simulink model "six_step_inverter"  (R2023b)
settings: Solver=VariableStepAuto  StartTime=0.0  StopTime=2  RelTol=1e-3
libraries: spsIGBTDiodeLib x6, spsSeriesRLCBranchLib x3, spsDCVoltageSourceLib x1, spsGroundLib x1, spsMultimeterLib x1, sps_lib x1
settings Model: Creator=lmanglicmot  LastModifiedBy=lmanglicmot
settings DataIOCC: ReturnWorkspaceOutputs=off
settings OptimizationCC: ReuseModelBlockBuffer=off

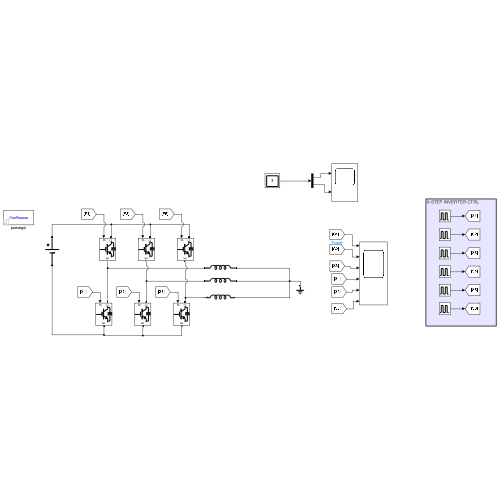
[thumbnail: Simulink's stored preview of the top-level diagram]
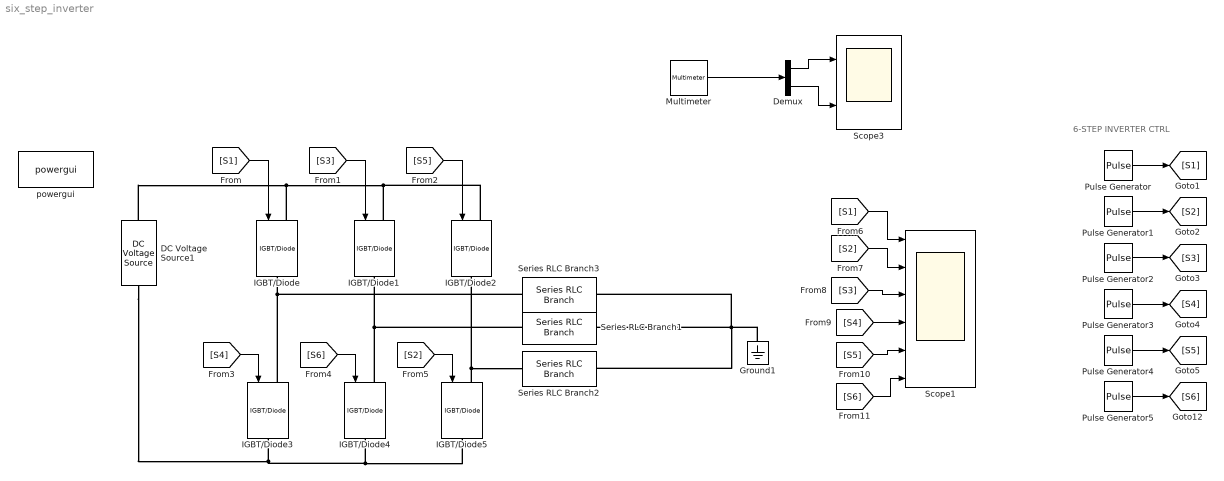
== system six_step_inverter ==
  note: 6-STEP INVERTER CTRL
  DC Voltage Source1 : spsDCVoltageSourceLib/DC Voltage Source  Amplitude=50  Measurements=None
  Demux : Demux  Outputs=2
  Ground1 : spsGroundLib/Ground  LConnTagsString=a
  IGBT/Diode{,1..5} (6 alike) : spsIGBTDiodeLib/IGBT//Diode  Ron=1e-3  Rs=1e5  Cs=inf  Measurements=off
  Multimeter : spsMultimeterLib/Multimeter  L=3  sel=[1 2 3]  yselected={}  Gain=[1 1 1]  OutputType=Complex  PlotAtSimulationStop=off  PhasorSimulation=off
  Pulse Generator : DiscretePulseGenerator  PulseType=Time based  Period=1/60  PulseWidth=50%
  Pulse Generator1 : DiscretePulseGenerator  PulseType=Time based  Period=1/60  PulseWidth=50%  PhaseDelay=(1/6)*1/60
  Pulse Generator2 : DiscretePulseGenerator  PulseType=Time based  Period=1/60  PulseWidth=50%  PhaseDelay=(2/6)*1/60
  Pulse Generator3 : DiscretePulseGenerator  PulseType=Time based  Period=1/60  PulseWidth=50  PhaseDelay=(3/6)*1/60
  Pulse Generator4 : DiscretePulseGenerator  PulseType=Time based  Period=1/60  PulseWidth=50%  PhaseDelay=(4/6)*1/60
  Pulse Generator5 : DiscretePulseGenerator  PulseType=Time based  Period=1/60  PulseWidth=50%  PhaseDelay=(5/6)*1/60
  Scope1 : Scope  NumInputPorts=6
  Scope3 : Scope  NumInputPorts=2
  Series RLC Branch1 : spsSeriesRLCBranchLib/Series RLC Branch  LConnTagsString=__new0  RConnTagsString=__new0  BranchType=L  Resistance=1  Inductance=5e-3  SetiL0=off  InitialCurrent=0  Capacitance=1e-6  Setx0=off  InitialVoltage=0  Measurements=Branch voltage
  Series RLC Branch2 : spsSeriesRLCBranchLib/Series RLC Branch  LConnTagsString=__new0  RConnTagsString=__new0  BranchType=L  Resistance=1  Inductance=5e-3  SetiL0=off  InitialCurrent=0  Capacitance=1e-6  Setx0=off  InitialVoltage=0  Measurements=Branch voltage
  Series RLC Branch3 : spsSeriesRLCBranchLib/Series RLC Branch  LConnTagsString=__new0  RConnTagsString=__new0  BranchType=L  Resistance=1  Inductance=5e-3  SetiL0=off  InitialCurrent=0  Capacitance=1e-6  Setx0=off  InitialVoltage=0  Measurements=Branch voltage
  powergui : sps_lib/powergui  Priority=1  SimulationMode=Continuous  SampleTime=1e-6  frequency=60  Iterations=50  frequencyindice=0  Pbase=100e6  ErrMax=1e-4  UnitsV=kV  UnitsW=MW  buscounter=0  FunctionMessages=off  echomessages=off  EnableUseOfTLC=off  CurrentSourceSwitches=off  DisableSnubberDevices=off  DisableRonSwitches=off  DisableVfSwitches=off  DisplayEquations=off  AutomaticDiscreteSolvers=off  SolverType=Tustin/Backward Euler (TBE)  Interpol=off  ExternalGateDelay=off  methode=off  Ts=100  x0status=blocks  SPID=on  SwTol=0  HookPort=off  NonlinearTolerance=1e-4  nMaxIteration=100  ContinueOnMaxIteration=off  RestoreLinks=warning  ResistiveCurrentMeasurement=off  Frange=[0:2:500]  Ylog=off  Xlog=on  ShowGrid=off  save=off  variable=ZData  structure=0  ZoomFFT=off  StartTime=0.0  cycles=1  DisplayStyle=1  fundamental=60  FreqAxis=off  MaxFrequency=1000  frequencyindicesteady=1  RmsSteady=1  display=off
  wires:
  [S1] -> IGBT/Diode/1
  [S3] -> IGBT/Diode1/1
  [S5] -> IGBT/Diode2/1
  [S4] -> IGBT/Diode3/1
  [S6] -> IGBT/Diode4/1
  [S2] -> IGBT/Diode5/1
  Pulse Generator/1 -> [S1]
  Pulse Generator1/1 -> [S2]
  Pulse Generator2/1 -> [S3]
  Pulse Generator3/1 -> [S4]
  Pulse Generator4/1 -> [S5]
  Pulse Generator5/1 -> [S6]
  [S1] -> Scope1/1
  [S2] -> Scope1/2
  [S3] -> Scope1/3
  [S4] -> Scope1/4
  [S5] -> Scope1/5
  [S6] -> Scope1/6
  Multimeter/1 -> Demux/1
  Demux/1 -> Scope3/1
  Demux/2 -> Scope3/2
  connections:
  Series RLC Branch3/LConn1 -- IGBT/Diode/RConn1 -- IGBT/Diode3/LConn1
  IGBT/Diode4/LConn1 -- IGBT/Diode1/RConn1 -- Series RLC Branch1/LConn1
  IGBT/Diode5/LConn1 -- IGBT/Diode2/RConn1 -- Series RLC Branch2/LConn1
  IGBT/Diode/LConn1 -- DC Voltage Source1/RConn1 -- IGBT/Diode2/LConn1 -- IGBT/Diode1/LConn1
  IGBT/Diode5/RConn1 -- DC Voltage Source1/LConn1 -- IGBT/Diode3/RConn1 -- IGBT/Diode4/RConn1
  Ground1/LConn1 -- Series RLC Branch2/RConn1 -- Series RLC Branch1/RConn1 -- Series RLC Branch3/RConn1
